simulink model "temp_rst_controller"  (Simulink 4.00)
settings: Solver=FixedStepDiscrete  StartTime=0.0  StopTime=160  FixedStep=0.05  RelTol=1e-3
libraries: rst_controller_lib x2
settings Model: LastModifiedBy=bsaunder

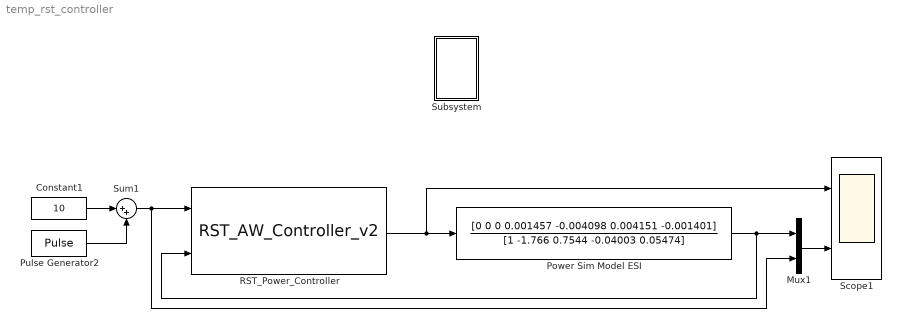
== system temp_rst_controller ==
  Constant1 : Constant  Value=10
  Mux1 : Mux  Inputs=2
  Power Sim Model ESI : DiscreteFilter  Numerator=[0 0 0 0.001457 -0.004098 0.004151 -0.001401]  Denominator=[1 -1.766 0.7544 -0.04003 0.05474]  SampleTime=0.05  Realization=auto
      settings: RTWStateStorageClass=Auto
  Pulse Generator2 : DiscretePulseGenerator  PulseType=Time-based  Amplitude=5  Period=40  PulseWidth=50  PhaseDelay=0  SampleTime=1
  RST_Power_Controller : rst_controller_lib/RST_AW_Controller_v2  out_limit=[0 500]
  Scope1 : Scope  NumInputPorts=2
      settings: TimeRange=160  YMin=0~-2  YMax=450~16  SaveToWorkspace=off  LimitDataPoints=on  MaxDataPoints=5000
  Subsystem : Subsystem
      settings: RTWFcnNameOpts=Auto  RTWFileNameOpts=Auto
  Sum1 : Sum  Inputs=|++  SaturateOnIntegerOverflow=on
  wires:
  Constant1/1 -> Sum1/1
  Pulse Generator2/1 -> Sum1/2
  Sum1/1 -> Mux1/2, RST_Power_Controller/1
  RST_Power_Controller/1 -> Scope1/1, Power Sim Model ESI/1
  Power Sim Model ESI/1 -> Mux1/1, RST_Power_Controller/2
  Mux1/1 -> Scope1/2

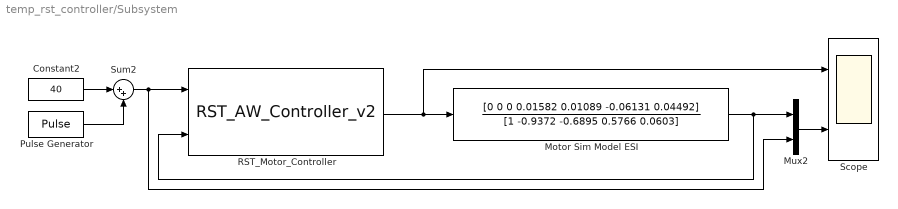
== system temp_rst_controller/Subsystem ==
  Constant2 : Constant  Value=40
  Motor Sim Model ESI : DiscreteFilter  Numerator=[0 0 0 0.01582 0.01089 -0.06131 0.04492]  Denominator=[1 -0.9372 -0.6895 0.5766 0.0603]  SampleTime=0.05  Realization=auto
      settings: RTWStateStorageClass=Auto
  Mux2 : Mux  Inputs=2
  Pulse Generator : DiscretePulseGenerator  PulseType=Time-based  Amplitude=20  Period=40  PulseWidth=50  PhaseDelay=0  SampleTime=1
  RST_Motor_Controller : rst_controller_lib/RST_AW_Controller_v2  out_limit=[0 100]
  Scope : Scope  NumInputPorts=2
      settings: TimeRange=160  YMin=0~0  YMax=70~70  SaveToWorkspace=off  SaveName=ScopeData  LimitDataPoints=on  MaxDataPoints=5000
  Sum2 : Sum  Inputs=|++  SaturateOnIntegerOverflow=on
  wires:
  Constant2/1 -> Sum2/1
  Pulse Generator/1 -> Sum2/2
  Sum2/1 -> Mux2/2, RST_Motor_Controller/1
  RST_Motor_Controller/1 -> Scope/1, Motor Sim Model ESI/1
  Motor Sim Model ESI/1 -> Mux2/1, RST_Motor_Controller/2
  Mux2/1 -> Scope/2
